simulink model "PathSignal"  (R2025a)
settings: Solver=FixedStepAuto  StartTime=0.0  StopTime=10.0  FixedStep=0.01  RelTol=1e-3
libraries: simulink x2
settings Model: Creator=levirogalla  LastModifiedBy=levirogalla

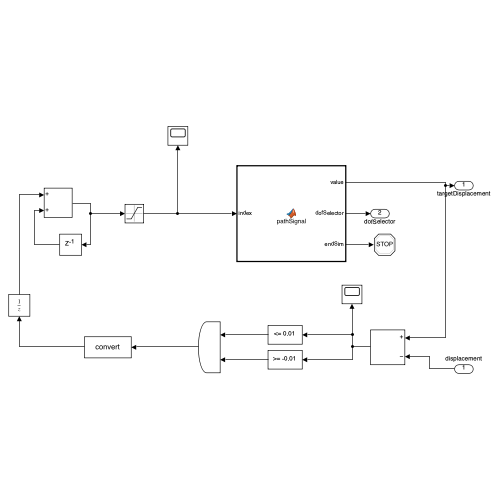
[thumbnail: Simulink's stored preview of the top-level diagram]
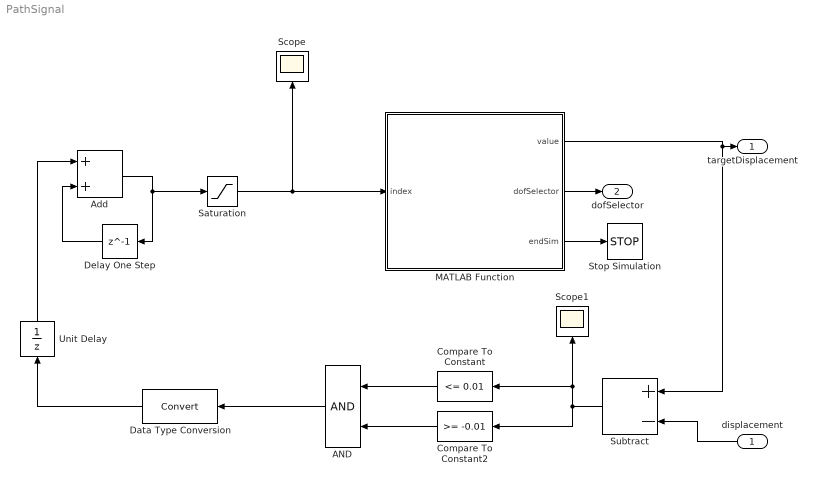
== system PathSignal ==
  displacement : Inport
  AND : Logic  IconShape=distinctive  AllPortsSameDT=off  OutDataTypeStr=boolean
  Add : Sum
  Compare To Constant : simulink/Logic and Bit Operations/Compare To Constant  relop=<=  const=0.01  OutDataTypeStr=boolean
  Compare To Constant2 : simulink/Logic and Bit Operations/Compare To Constant  relop=>=  const=-0.01  OutDataTypeStr=boolean
  Data Type Conversion : DataTypeConversion  SaturateOnIntegerOverflow=off  RndMeth=Floor
  Delay One Step : Delay  DelayLength=1
  MATLAB Function : MATLAB Function  TreatAsAtomicUnit=on
  Saturation : Saturate  UpperLimit=5  LowerLimit=0  LinearizeAsGain=off
  Scope : Scope
      settings: ActiveDisplayYMinimum=-0.125  ActiveDisplayYMaximum=1.125
  Scope1 : Scope
      settings: ActiveDisplayYMinimum=-1.2066542764324755  ActiveDisplayYMaximum=1.5069367792859989  DataLoggingVariableName=ScopeData2
  Stop Simulation : Stop
  Subtract : Sum  Inputs=+-
  Unit Delay : UnitDelay  SampleTime=-1  HasFrameUpgradeWarning=on
  targetDisplacement : Outport
  dofSelector : Outport  Port=2
  wires:
  Delay One Step/1 -> Add/2
  Unit Delay/1 -> Add/1
  AND/1 -> Data Type Conversion/1
  Compare To Constant2/1 -> AND/2
  Subtract/1 -> Compare To Constant2/1, Scope1/1, Compare To Constant/1
  Compare To Constant/1 -> AND/1
  MATLAB Function/3(endSim) -> Stop Simulation/1
  MATLAB Function/1(value) -> targetDisplacement/1, Subtract/1
  Add/1 -> Delay One Step/1, Saturation/1
  Saturation/1 -> MATLAB Function/1(index), Scope/1
  Data Type Conversion/1 -> Unit Delay/1
  MATLAB Function/2(dofSelector) -> dofSelector/1
  displacement/1 -> Subtract/2

== matlab function PathSignal/MATLAB Function ==
  data: value output; dofSelector output; index input; endSim output
function [value, dofSelector, endSim] = pathSignal(index)
% Returns path values and a signal to stop simulation when out of bounds

% Define the path matrix
pathMatrix = [15, 1;
             -pi/2, 3;
             -10.1, 2;
             -pi, 3;
              6.9, 1
              -pi, 3];

% Get the size of the path
N = size(pathMatrix, 1);

% Initialize outputs
value = 0;
dofSelector = 1;
endSim = false;

% Check if index is within bounds
if index + 1 <= N
    value = pathMatrix(index + 1, 1);
    dofSelector = pathMatrix(index + 1, 2);
else
    endSim = true;  % signal to stop the simulation
end
